simulink model "pi_dam_water_level"  (R2026a)
settings: Solver=ode45  StopTime=1000
undefined symbols (not defined in the file): p
settings Model: Creator=mohamedelwalidfadul  LastModifiedBy=mohamedelwalidfadul

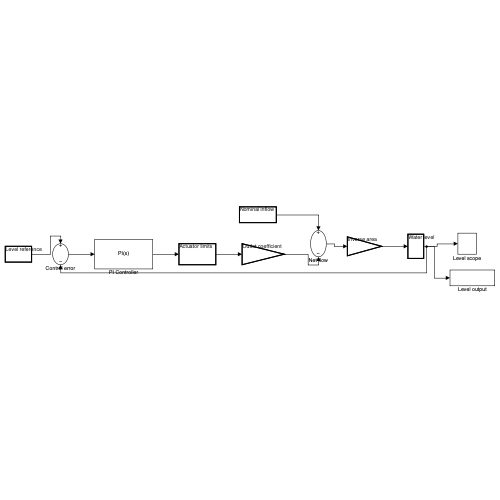
[thumbnail: Simulink's stored preview of the top-level diagram]
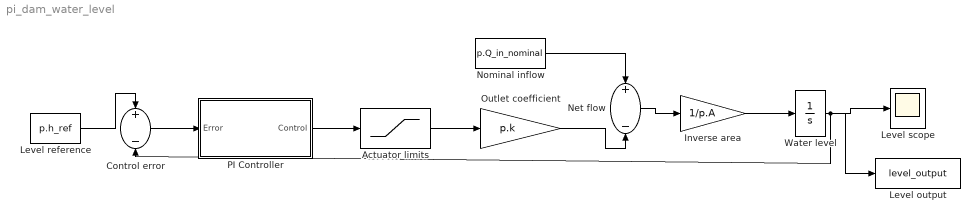
== system pi_dam_water_level ==
  Actuator limits : Saturate  UpperLimit=p.u_max  LowerLimit=p.u_min
  Control error : Sum  Inputs=+-
  Inverse area : Gain  Gain=1/p.A
  Level output : ToWorkspace  VariableName=level_output  SaveFormat=Structure With Time  SampleTime=-1
  Level reference : Constant  Value=p.h_ref
  Level scope : Scope
  Net flow : Sum  Inputs=+-
  Nominal inflow : Constant  Value=p.Q_in_nominal
  Outlet coefficient : Gain  Gain=p.k
  PI Controller : Subsystem
      mask Display: disp('PI(s)')
  Water level : Integrator  InitialCondition=p.h_initial
  wires:
  Level reference/1 -> Control error/1
  Control error/1 -> PI Controller/1(Error)
  PI Controller/1(Control) -> Actuator limits/1
  Actuator limits/1 -> Outlet coefficient/1
  Nominal inflow/1 -> Net flow/1
  Outlet coefficient/1 -> Net flow/2
  Net flow/1 -> Inverse area/1
  Inverse area/1 -> Water level/1
  Water level/1 -> Level scope/1, Level output/1, Control error/2

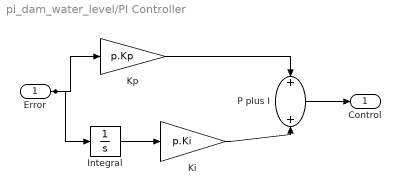
== system pi_dam_water_level/PI Controller ==
  Error : Inport
  Integral : Integrator
  Ki : Gain  Gain=p.Ki
  Kp : Gain  Gain=p.Kp
  P plus I : Sum
  Control : Outport
  wires:
  Error/1 -> Kp/1, Integral/1
  Kp/1 -> P plus I/1
  Integral/1 -> Ki/1
  Ki/1 -> P plus I/2
  P plus I/1 -> Control/1
